simulink model "halbwegs_funktionierend_EinAusgangsLinearisierung"  (R2024b)
settings: Solver=VariableStepAuto  StartTime=0.0  StopTime=10
InitFcn:
  | R = 1e+3;
  | L = 100e-3;
  | C1 = 100e-9;
  | C2 = 1e-6;
  | 
  | k  = 1.380649e-23;
  | e  = 1.602176634e-19;
  | T  = 25 + 273.15;
  | UT = k*T/e;
  | IS = 10e-9;
  | 
  | U0 = 12;
  | I0 = 10e-3;
  | 
  | syms U1 U2 IL
  | x = [U1, U2, IL];
  | %Zerlegung in System-, Ausgangs- und Eingangswirkung
  | f_ea = [
  |     -IS*exp(-U2/UT)/C1 + IL/C1;
  |     IL/C2;
  |     -U1/L - U2/L - R*IL/L
  | ]
  | g_ea = [
  |     0, 0;
  |     0, -1/C2;
  |     1/L, 0;
  | ]
  | g_ea_U0 = [
  |     0;
  |     0;
  |     1/L;
  | ]
  | g_ea_I0 = [
  |     0;
  |     -1/C2;
  |     0;
  | ]
  | h_ea = U2 %for y = xi set h_ea at position i to 1
  | h_ea_simulink = gradient(h_ea, x)
  | %Lie-Ableitungen berechnen
  | Lf = h_ea;
  | Lf_h = Lf;
  | r = 0;
  | 
  | Lf_r_init = sym(zeros(10,1))
  | Lf_r_init(1) = Lf_h
  | 
  | 
  | while true
  |     LgLf = jacobian(Lf, x) * g_ea % x = [U1; U2; IL]
  |     if (LgLf(1) ~= 0 || LgLf(2) ~= 0)
  |         % vermutlich notwendig, um L_f^r h anstelle von L_f^{(r-1)} h zu
  |         % erhalten
  |         Lf = jacobian(Lf, x) * f_ea
  |         Lf_h = Lf
  |         %
  |         break;
  |     end
  |     Lf = jacobian(Lf, x) * f_ea % x = [U1; U2; IL], Lf = IL/C2
  |     Lf_h = Lf
  |     Lf_r_init(r+2) = Lf_h
  |     r = r + 1
  | end
  | 
  | r = r + 1
  | 
  | if r == 1
  |     Lf_r = zeros(1,1);
  |     Lf_r = Lf_r_init(1);
  | 
  |     % Pole für Regelung:
  |     p = [-3];
  | end
  | 
  | if r == 2
  |     Lf_r = zeros(2,1);
  |     Lf_r = Lf_r_init(1);
  |     Lf_r = Lf_r_init(2);
  | 
  |     % Pole für Regelung:
  |     p = [-2-2*i, -2+2*i];
  | end
  | 
  | phi = Lf_r
  | 
  | syms v
  | L_nom = v - Lf_h % letzte Lf
  | L_denom = LgLf
  | 
  | 
  | 
  | L_script = L_nom * pinv(L_denom)
  | L_pinv = pinv(L_denom)
  | 
  | alpha = LgLf
  | beta = Lf_h
  | 
  | 
  | 
  | %%%A-, B-, und C-Matrix
  | A = zeros(r);
  | for i=1:r
  |     for j=1:r
  |         if j == i+1
  |             A(i,j) = 1;
  |         end
  |     end
  | end
  | A
  | %%Oder:
  | %A = diag(ones(r-1,1), 1);
  | 
  | B = zeros(r,1);
  | B(r) = 1
  | 
  | C = zeros(1,r);
  | C(1) = 1
  | 
  | %syms U2_ref Kp
  | %v = Kp * (U2_ref - U2);
  | 
  | G = place(A, B, p)
  | 
  | disp(LgLf)
  | disp(Lf_h)
  | LfLg_pinv = pinv(LgLf)
  | disp(LfLg_pinv);
settings Model: Creator=richa  LastModifiedBy=richa
settings ConfigComp: CovBoundaryAbsTol=1.0e-5

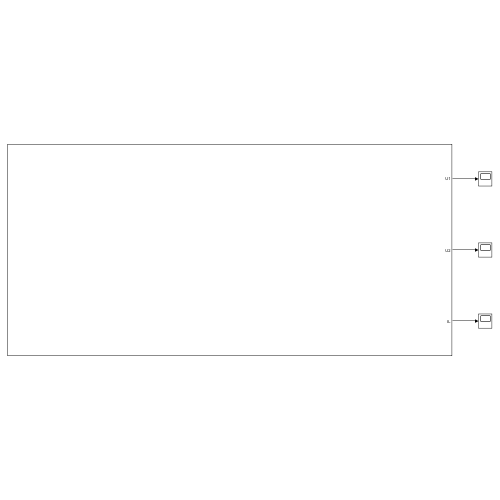
[thumbnail: Simulink's stored preview of the top-level diagram]
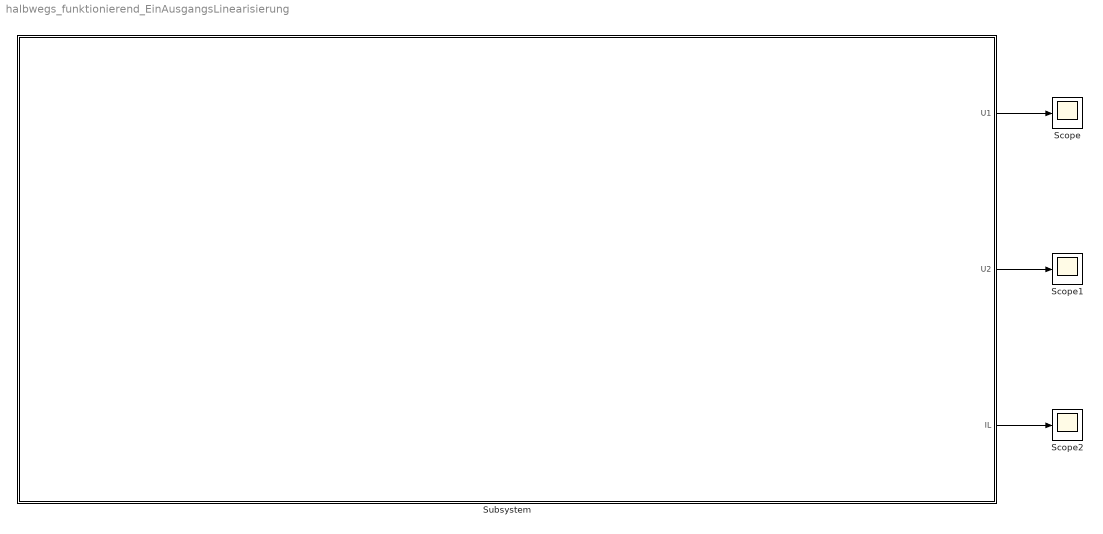
== system halbwegs_funktionierend_EinAusgangsLinearisierung ==
  Scope : Scope
  Scope1 : Scope
  Scope2 : Scope
  Subsystem : Subsystem
  wires:
  Subsystem/1(U1) -> Scope/1
  Subsystem/2(U2) -> Scope1/1
  Subsystem/3(IL) -> Scope2/1

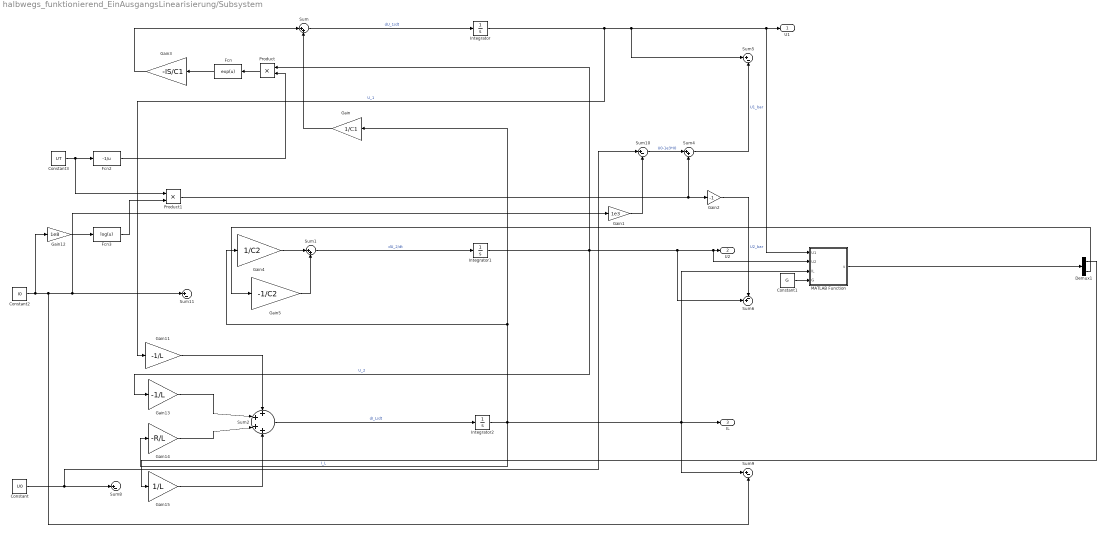
== system halbwegs_funktionierend_EinAusgangsLinearisierung/Subsystem ==
  Constant : Constant  Value=U0
  Constant1 : Constant  Value=G
  Constant2 : Constant  Value=I0
  Constant3 : Constant  Value=UT
  Demux1 : Demux  Outputs=2
  Fcn : Fcn  Expr=exp(u)
  Fcn2 : Fcn  Expr=-1/u
  Fcn3 : Fcn  Expr=log(u)
  Gain : Gain  Gain=1/C1
  Gain1 : Gain  Gain=1e3
  Gain11 : Gain  Gain=-1/L
  Gain12 : Gain  Gain=1e8
  Gain13 : Gain  Gain=-1/L
  Gain14 : Gain  Gain=-R/L
  Gain15 : Gain  Gain=1/L
  Gain2 : Gain  Gain=-1
  Gain3 : Gain  Gain=-IS/C1
  Gain4 : Gain  Gain=1/C2
  Gain5 : Gain  Gain=-1/C2
  Integrator : Integrator
  Integrator1 : Integrator
  Integrator2 : Integrator
  MATLAB Function : MATLAB Function  TreatAsAtomicUnit=on
  Product : Product
  Product1 : Product
  Sum : Sum  Inputs=|++
  Sum1 : Sum  Inputs=|++
  Sum{5,8..11} (5 alike) : Sum  Inputs=|+-
  Sum2 : Sum  Inputs=++++
  Sum4 : Sum  Inputs=|++
  Sum6 : Sum  Inputs=-+|
  U1 : Outport
  U2 : Outport  Port=2
  IL : Outport  Port=3
  wires:
  Fcn3/1 -> Product1/2
  Gain4/1 -> Sum1/1
  Gain11/1 -> Sum2/1
  Constant/1 -> Sum8/1, Sum10/1
  Fcn2/1 -> Product/2
  Gain/1 -> Sum/2
  Gain1/1 -> Sum10/2
  Gain12/1 -> Fcn3/1
  Gain13/1 -> Sum2/2
  Gain5/1 -> Sum1/2
  Integrator1/1 -> MATLAB Function/2(U2), U2/1, Sum6/2, Product/1, Gain13/1  "U_2"
  Gain3/1 -> Sum/1
  Sum1/1 -> Integrator1/1  "dU_2/dt"
  Sum4/1 -> Sum5/2  "U1_bar"
  Constant2/1 -> Gain12/1, Sum11/1, Gain1/1, Sum9/2
  Integrator/1 -> MATLAB Function/1(U1), U1/1, Sum5/1, Gain11/1  "U_1"
  Constant3/1 -> Product1/1, Fcn2/1
  Product/1 -> Fcn/1
  Gain14/1 -> Sum2/3
  Product1/1 -> Gain2/1, Sum4/2
  Sum/1 -> Integrator/1  "dU_1/dt"
  Sum10/1 -> Sum4/1  "U0-1e3*I0"
  Fcn/1 -> Gain3/1
  Gain15/1 -> Sum2/4
  Sum2/1 -> Integrator2/1  "dI_L/dt"
  Integrator2/1 -> MATLAB Function/3(IL), Sum9/1, IL/1, Gain14/1, Gain/1, Gain4/1  "I_L"
  Gain2/1 -> Sum6/1  "U2_bar"
  Demux1/1 -> Gain15/1
  Demux1/2 -> Gain5/1
  MATLAB Function/1(u) -> Demux1/1
  Constant1/1 -> MATLAB Function/4(G)

== matlab function halbwegs_funktionierend_EinAusgangsLinearisierung/Subsystem/MATLAB Function ==
  data: U1 input; u output; U2 input; IL input; G input
function u = fcn(U1, U2, IL, G)

    z = U2;

    v = -G*(z - 10);
    
    % u = alpha^-1 * (v - beta)
    u = [0; -1/1000000] * (v + 1000000*IL);

end
